simulink model "Roadsense_ScenarioClosedLoopHarness"  (R2025b)
settings: Solver=FixedStepDiscrete  StartTime=0.0  StopTime=25  FixedStep=RsTsBase  RelTol=1e-3
undefined symbols (not defined in the file or in its folder): RsTsBase, RsTsControl, RsTsScenario
settings Model: DataDictionary=Roadsense_Data.sldd  Creator=ragur  LastModifiedBy=ragur

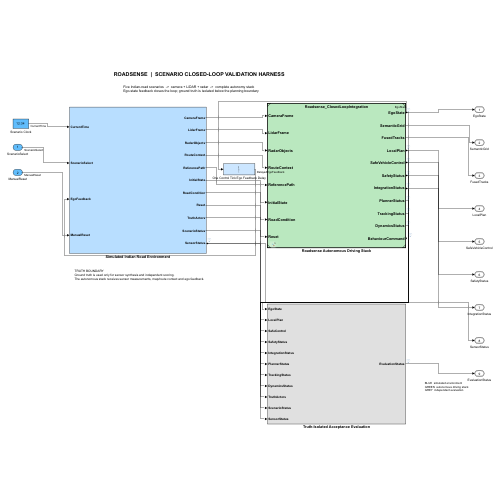
[thumbnail: Simulink's stored preview of the top-level diagram]
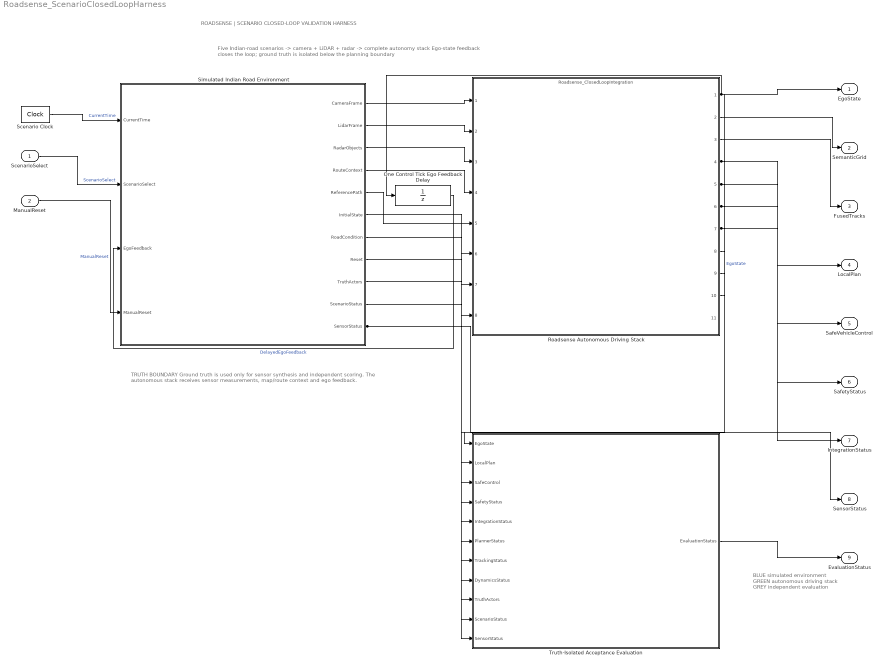
== system Roadsense_ScenarioClosedLoopHarness ==
  note: ROADSENSE | SCENARIO CLOSED-LOOP VALIDATION HARNESS
  note: Five Indian-road scenarios  ->  camera + LiDAR + radar  ->  complete autonomy stack
      | Ego-state feedback closes the loop; ground truth is isolated below the planning boundary
  note: TRUTH BOUNDARY
      | Ground truth is used only for sensor synthesis and independent scoring.
      | The autonomous stack receives sensor measurements, map/route context and ego feedback.
  note: BLUE  simulated environment
      | GREEN  autonomous driving stack
      | GREY  independent evaluation
  ScenarioSelect : Inport  OutDataTypeStr=uint8  SampleTime=RsTsScenario
  ManualReset : Inport  Port=2  OutDataTypeStr=boolean  SampleTime=RsTsControl
  One Control Tick Ego Feedback Delay : UnitDelay  SampleTime=RsTsControl  HasFrameUpgradeWarning=on
  Roadsense Autonomous Driving Stack : ModelReference  ModelNameDialog=Roadsense_ClosedLoopIntegration  SimulationMode=Normal  ModelReferenceVersion=1.1
  Scenario Clock : DigitalClock  SampleTime=RsTsBase
  Simulated Indian Road Environment : Subsystem
  Truth-Isolated Acceptance Evaluation : Subsystem
  EgoState : Outport  OutDataTypeStr=Bus: RsEgoStateBus
  SemanticGrid : Outport  Port=2  OutDataTypeStr=Bus: RsSemanticGridBus
  FusedTracks : Outport  Port=3  OutDataTypeStr=Bus: RsFusedTrackListBus
  LocalPlan : Outport  Port=4  OutDataTypeStr=Bus: RsLocalPlanBus
  SafeVehicleControl : Outport  Port=5  OutDataTypeStr=Bus: RsVehicleControlBus
  SafetyStatus : Outport  Port=6  OutDataTypeStr=Bus: RsSafetyStatusBus
  IntegrationStatus : Outport  Port=7  OutDataTypeStr=Bus: RsIntegrationStatusBus
  SensorStatus : Outport  Port=8  OutDataTypeStr=Bus: RsScenarioSensorStatusBus
  EvaluationStatus : Outport  Port=9  OutDataTypeStr=Bus: RsScenarioEvaluationBus
  wires:
  Scenario Clock/1 -> Simulated Indian Road Environment/1(CurrentTime)  "CurrentTime"
  ScenarioSelect/1 -> Simulated Indian Road Environment/2(ScenarioSelect)  "ScenarioSelect"
  Roadsense Autonomous Driving Stack/1 -> One Control Tick Ego Feedback Delay/1, Truth-Isolated Acceptance Evaluation/1(EgoState), EgoState/1  "EgoState"
  One Control Tick Ego Feedback Delay/1 -> Simulated Indian Road Environment/3(EgoFeedback)  "DelayedEgoFeedback"
  ManualReset/1 -> Simulated Indian Road Environment/4(ManualReset)  "ManualReset"
  Simulated Indian Road Environment/1(CameraFrame) -> Roadsense Autonomous Driving Stack/1
  Simulated Indian Road Environment/2(LidarFrame) -> Roadsense Autonomous Driving Stack/2
  Simulated Indian Road Environment/3(RadarObjects) -> Roadsense Autonomous Driving Stack/3
  Simulated Indian Road Environment/4(RouteContext) -> Roadsense Autonomous Driving Stack/4
  Simulated Indian Road Environment/5(ReferencePath) -> Roadsense Autonomous Driving Stack/5
  Simulated Indian Road Environment/6(InitialState) -> Roadsense Autonomous Driving Stack/6
  Simulated Indian Road Environment/7(RoadCondition) -> Roadsense Autonomous Driving Stack/7
  Simulated Indian Road Environment/8(Reset) -> Roadsense Autonomous Driving Stack/8
  Roadsense Autonomous Driving Stack/4 -> Truth-Isolated Acceptance Evaluation/2(LocalPlan), LocalPlan/1
  Roadsense Autonomous Driving Stack/5 -> Truth-Isolated Acceptance Evaluation/3(SafeControl), SafeVehicleControl/1
  Roadsense Autonomous Driving Stack/6 -> Truth-Isolated Acceptance Evaluation/4(SafetyStatus), SafetyStatus/1
  Roadsense Autonomous Driving Stack/7 -> Truth-Isolated Acceptance Evaluation/5(IntegrationStatus), IntegrationStatus/1
  Roadsense Autonomous Driving Stack/8 -> Truth-Isolated Acceptance Evaluation/6(PlannerStatus)
  Roadsense Autonomous Driving Stack/9 -> Truth-Isolated Acceptance Evaluation/7(TrackingStatus)
  Roadsense Autonomous Driving Stack/10 -> Truth-Isolated Acceptance Evaluation/8(DynamicsStatus)
  Simulated Indian Road Environment/9(TruthActors) -> Truth-Isolated Acceptance Evaluation/9(TruthActors)
  Simulated Indian Road Environment/10(ScenarioStatus) -> Truth-Isolated Acceptance Evaluation/10(ScenarioStatus)
  Simulated Indian Road Environment/11(SensorStatus) -> Truth-Isolated Acceptance Evaluation/11(SensorStatus), SensorStatus/1
  Roadsense Autonomous Driving Stack/2 -> SemanticGrid/1
  Roadsense Autonomous Driving Stack/3 -> FusedTracks/1
  Truth-Isolated Acceptance Evaluation/1(EvaluationStatus) -> EvaluationStatus/1

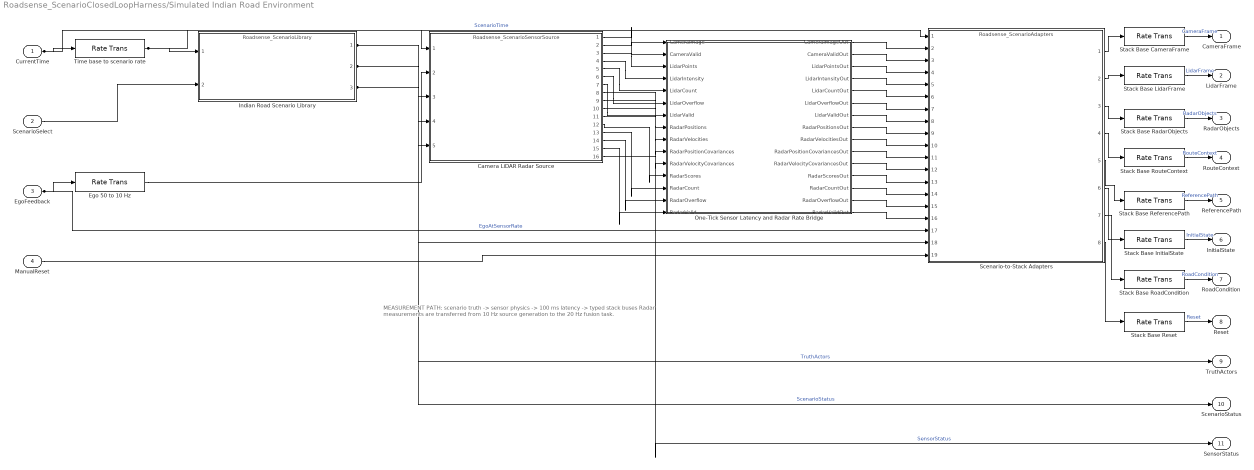
== system Roadsense_ScenarioClosedLoopHarness/Simulated Indian Road Environment ==
  note: MEASUREMENT PATH:  scenario truth -> sensor physics -> 100 ms latency -> typed stack buses
      | Radar measurements are transferred from 10 Hz source generation to the 20 Hz fusion task.
  CurrentTime : Inport  OutDataTypeStr=double  SampleTime=RsTsBase
  ScenarioSelect : Inport  Port=2  OutDataTypeStr=uint8  SampleTime=RsTsScenario
  EgoFeedback : Inport  Port=3  OutDataTypeStr=Bus: RsEgoStateBus  SampleTime=RsTsControl
  ManualReset : Inport  Port=4  OutDataTypeStr=boolean  SampleTime=RsTsControl
  Camera LiDAR Radar Source : ModelReference  ModelNameDialog=Roadsense_ScenarioSensorSource  SimulationMode=Normal  ModelReferenceVersion=1.1
  Ego 50 to 10 Hz : RateTransition  OutPortSampleTime=RsTsScenario
  Indian Road Scenario Library : ModelReference  ModelNameDialog=Roadsense_ScenarioLibrary  SimulationMode=Normal  ModelReferenceVersion=1.1
  One-Tick Sensor Latency and Radar Rate Bridge : Subsystem
  Scenario-to-Stack Adapters : ModelReference  ModelNameDialog=Roadsense_ScenarioAdapters  SimulationMode=Normal  ModelReferenceVersion=1.1
  Stack Base CameraFrame : RateTransition  OutPortSampleTime=RsTsBase
  Stack Base InitialState : RateTransition  OutPortSampleTime=RsTsBase
  Stack Base LidarFrame : RateTransition  OutPortSampleTime=RsTsBase
  Stack Base RadarObjects : RateTransition  OutPortSampleTime=RsTsBase
  Stack Base ReferencePath : RateTransition  OutPortSampleTime=RsTsBase
  Stack Base Reset : RateTransition  OutPortSampleTime=RsTsBase
  Stack Base RoadCondition : RateTransition  OutPortSampleTime=RsTsBase
  Stack Base RouteContext : RateTransition  OutPortSampleTime=RsTsBase
  Time base to scenario rate : RateTransition  OutPortSampleTime=RsTsScenario
  CameraFrame : Outport  OutDataTypeStr=Bus: RsCameraFrameBus
  LidarFrame : Outport  Port=2  OutDataTypeStr=Bus: RsLidarFrameBus
  RadarObjects : Outport  Port=3  OutDataTypeStr=Bus: RsRadarObjectListBus
  RouteContext : Outport  Port=4  OutDataTypeStr=Bus: RsRouteContextBus
  ReferencePath : Outport  Port=5  OutDataTypeStr=Bus: RsReferencePathBus
  InitialState : Outport  Port=6  OutDataTypeStr=Bus: RsEgoStateBus
  RoadCondition : Outport  Port=7  OutDataTypeStr=Bus: RsRoadConditionBus
  Reset : Outport  Port=8  OutDataTypeStr=boolean
  TruthActors : Outport  Port=9  OutDataTypeStr=Bus: RsScenarioActorListBus
  ScenarioStatus : Outport  Port=10  OutDataTypeStr=Bus: RsScenarioStatusBus
  SensorStatus : Outport  Port=11  OutDataTypeStr=Bus: RsScenarioSensorStatusBus
  wires:
  CurrentTime/1 -> Time base to scenario rate/1, Scenario-to-Stack Adapters/1  "ScenarioTime"
  EgoFeedback/1 -> Ego 50 to 10 Hz/1, Scenario-to-Stack Adapters/17  "EgoAtSensorRate"
  Time base to scenario rate/1 -> Indian Road Scenario Library/1, Camera LiDAR Radar Source/1
  ScenarioSelect/1 -> Indian Road Scenario Library/2
  Ego 50 to 10 Hz/1 -> Camera LiDAR Radar Source/2
  Indian Road Scenario Library/2 -> Camera LiDAR Radar Source/3, TruthActors/1  "TruthActors"
  Indian Road Scenario Library/1 -> Camera LiDAR Radar Source/4, Scenario-to-Stack Adapters/18
  Indian Road Scenario Library/3 -> Camera LiDAR Radar Source/5, ScenarioStatus/1  "ScenarioStatus"
  Camera LiDAR Radar Source/1 -> One-Tick Sensor Latency and Radar Rate Bridge/1(CameraImage)
  Camera LiDAR Radar Source/2 -> One-Tick Sensor Latency and Radar Rate Bridge/2(CameraValid)
  Camera LiDAR Radar Source/3 -> One-Tick Sensor Latency and Radar Rate Bridge/3(LidarPoints)
  Camera LiDAR Radar Source/4 -> One-Tick Sensor Latency and Radar Rate Bridge/4(LidarIntensity)
  Camera LiDAR Radar Source/5 -> One-Tick Sensor Latency and Radar Rate Bridge/5(LidarCount)
  Camera LiDAR Radar Source/6 -> One-Tick Sensor Latency and Radar Rate Bridge/6(LidarOverflow)
  Camera LiDAR Radar Source/7 -> One-Tick Sensor Latency and Radar Rate Bridge/7(LidarValid)
  Camera LiDAR Radar Source/8 -> One-Tick Sensor Latency and Radar Rate Bridge/8(RadarPositions)
  Camera LiDAR Radar Source/9 -> One-Tick Sensor Latency and Radar Rate Bridge/9(RadarVelocities)
  Camera LiDAR Radar Source/10 -> One-Tick Sensor Latency and Radar Rate Bridge/10(RadarPositionCovariances)
  Camera LiDAR Radar Source/11 -> One-Tick Sensor Latency and Radar Rate Bridge/11(RadarVelocityCovariances)
  Camera LiDAR Radar Source/12 -> One-Tick Sensor Latency and Radar Rate Bridge/12(RadarScores)
  Camera LiDAR Radar Source/13 -> One-Tick Sensor Latency and Radar Rate Bridge/13(RadarCount)
  Camera LiDAR Radar Source/14 -> One-Tick Sensor Latency and Radar Rate Bridge/14(RadarOverflow)
  Camera LiDAR Radar Source/15 -> One-Tick Sensor Latency and Radar Rate Bridge/15(RadarValid)
  One-Tick Sensor Latency and Radar Rate Bridge/1(CameraImageOut) -> Scenario-to-Stack Adapters/2
  One-Tick Sensor Latency and Radar Rate Bridge/2(CameraValidOut) -> Scenario-to-Stack Adapters/3
  One-Tick Sensor Latency and Radar Rate Bridge/3(LidarPointsOut) -> Scenario-to-Stack Adapters/4
  One-Tick Sensor Latency and Radar Rate Bridge/4(LidarIntensityOut) -> Scenario-to-Stack Adapters/5
  One-Tick Sensor Latency and Radar Rate Bridge/5(LidarCountOut) -> Scenario-to-Stack Adapters/6
  One-Tick Sensor Latency and Radar Rate Bridge/6(LidarOverflowOut) -> Scenario-to-Stack Adapters/7
  One-Tick Sensor Latency and Radar Rate Bridge/7(LidarValidOut) -> Scenario-to-Stack Adapters/8
  One-Tick Sensor Latency and Radar Rate Bridge/8(RadarPositionsOut) -> Scenario-to-Stack Adapters/9
  One-Tick Sensor Latency and Radar Rate Bridge/9(RadarVelocitiesOut) -> Scenario-to-Stack Adapters/10
  One-Tick Sensor Latency and Radar Rate Bridge/10(RadarPositionCovariancesOut) -> Scenario-to-Stack Adapters/11
  One-Tick Sensor Latency and Radar Rate Bridge/11(RadarVelocityCovariancesOut) -> Scenario-to-Stack Adapters/12
  One-Tick Sensor Latency and Radar Rate Bridge/12(RadarScoresOut) -> Scenario-to-Stack Adapters/13
  One-Tick Sensor Latency and Radar Rate Bridge/13(RadarCountOut) -> Scenario-to-Stack Adapters/14
  One-Tick Sensor Latency and Radar Rate Bridge/14(RadarOverflowOut) -> Scenario-to-Stack Adapters/15
  One-Tick Sensor Latency and Radar Rate Bridge/15(RadarValidOut) -> Scenario-to-Stack Adapters/16
  ManualReset/1 -> Scenario-to-Stack Adapters/19
  Scenario-to-Stack Adapters/1 -> Stack Base CameraFrame/1
  Stack Base CameraFrame/1 -> CameraFrame/1  "CameraFrame"
  Scenario-to-Stack Adapters/2 -> Stack Base LidarFrame/1
  Stack Base LidarFrame/1 -> LidarFrame/1  "LidarFrame"
  Scenario-to-Stack Adapters/3 -> Stack Base RadarObjects/1
  Stack Base RadarObjects/1 -> RadarObjects/1  "RadarObjects"
  Scenario-to-Stack Adapters/4 -> Stack Base RouteContext/1
  Stack Base RouteContext/1 -> RouteContext/1  "RouteContext"
  Scenario-to-Stack Adapters/5 -> Stack Base ReferencePath/1
  Stack Base ReferencePath/1 -> ReferencePath/1  "ReferencePath"
  Scenario-to-Stack Adapters/6 -> Stack Base InitialState/1
  Stack Base InitialState/1 -> InitialState/1  "InitialState"
  Scenario-to-Stack Adapters/7 -> Stack Base RoadCondition/1
  Stack Base RoadCondition/1 -> RoadCondition/1  "RoadCondition"
  Scenario-to-Stack Adapters/8 -> Stack Base Reset/1
  Stack Base Reset/1 -> Reset/1  "Reset"
  Camera LiDAR Radar Source/16 -> SensorStatus/1  "SensorStatus"

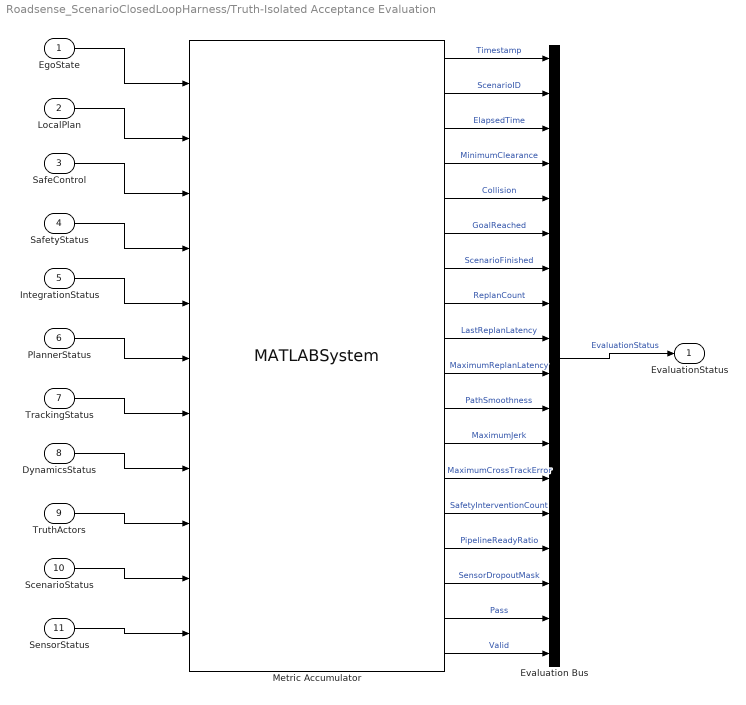
== system Roadsense_ScenarioClosedLoopHarness/Truth-Isolated Acceptance Evaluation ==
  EgoState : Inport  OutDataTypeStr=Bus: RsEgoStateBus
  LocalPlan : Inport  Port=2  OutDataTypeStr=Bus: RsLocalPlanBus
  SafeControl : Inport  Port=3  OutDataTypeStr=Bus: RsVehicleControlBus
  SafetyStatus : Inport  Port=4  OutDataTypeStr=Bus: RsSafetyStatusBus
  IntegrationStatus : Inport  Port=5  OutDataTypeStr=Bus: RsIntegrationStatusBus
  PlannerStatus : Inport  Port=6  OutDataTypeStr=Bus: RsPlannerStatusBus
  TrackingStatus : Inport  Port=7  OutDataTypeStr=Bus: RsTrackingStatusBus
  DynamicsStatus : Inport  Port=8  OutDataTypeStr=Bus: RsVehicleDynamicsStatusBus
  TruthActors : Inport  Port=9  OutDataTypeStr=Bus: RsScenarioActorListBus
  ScenarioStatus : Inport  Port=10  OutDataTypeStr=Bus: RsScenarioStatusBus
  SensorStatus : Inport  Port=11  OutDataTypeStr=Bus: RsScenarioSensorStatusBus
  Evaluation Bus : BusCreator  Inputs=18  OutDataTypeStr=Bus: RsScenarioEvaluationBus
  Metric Accumulator : MATLABSystem  System=RoadsenseScenarioEvaluationSystem  RequiredClearance=RsScenarioMinimumClearance  MaximumAllowedReplanLatency=RsScenarioMaximumReplanLatency  MaximumAllowedPathSmoothness=RsScenarioMaximumPathCurvatureRMS  MaximumAllowedJerk=RsScenarioMaximumJerk  MaximumAllowedCrossTrackError=RsScenarioMaximumCrossTrackError  MinimumReadyRatio=RsScenarioMinimumReadyRatio  SimulateUsing=Interpreted execution
      mask Type: RoadsenseScenarioEvaluationSystem
  EvaluationStatus : Outport  OutDataTypeStr=Bus: RsScenarioEvaluationBus
  wires:
  EgoState/1 -> Metric Accumulator/1
  LocalPlan/1 -> Metric Accumulator/2
  SafeControl/1 -> Metric Accumulator/3
  SafetyStatus/1 -> Metric Accumulator/4
  IntegrationStatus/1 -> Metric Accumulator/5
  PlannerStatus/1 -> Metric Accumulator/6
  TrackingStatus/1 -> Metric Accumulator/7
  DynamicsStatus/1 -> Metric Accumulator/8
  TruthActors/1 -> Metric Accumulator/9
  ScenarioStatus/1 -> Metric Accumulator/10
  SensorStatus/1 -> Metric Accumulator/11
  Metric Accumulator/1 -> Evaluation Bus/1  "Timestamp"
  Metric Accumulator/2 -> Evaluation Bus/2  "ScenarioID"
  Metric Accumulator/3 -> Evaluation Bus/3  "ElapsedTime"
  Metric Accumulator/4 -> Evaluation Bus/4  "MinimumClearance"
  Metric Accumulator/5 -> Evaluation Bus/5  "Collision"
  Metric Accumulator/6 -> Evaluation Bus/6  "GoalReached"
  Metric Accumulator/7 -> Evaluation Bus/7  "ScenarioFinished"
  Metric Accumulator/8 -> Evaluation Bus/8  "ReplanCount"
  Metric Accumulator/9 -> Evaluation Bus/9  "LastReplanLatency"
  Metric Accumulator/10 -> Evaluation Bus/10  "MaximumReplanLatency"
  Metric Accumulator/11 -> Evaluation Bus/11  "PathSmoothness"
  Metric Accumulator/12 -> Evaluation Bus/12  "MaximumJerk"
  Metric Accumulator/13 -> Evaluation Bus/13  "MaximumCrossTrackError"
  Metric Accumulator/14 -> Evaluation Bus/14  "SafetyInterventionCount"
  Metric Accumulator/15 -> Evaluation Bus/15  "PipelineReadyRatio"
  Metric Accumulator/16 -> Evaluation Bus/16  "SensorDropoutMask"
  Metric Accumulator/17 -> Evaluation Bus/17  "Pass"
  Metric Accumulator/18 -> Evaluation Bus/18  "Valid"
  Evaluation Bus/1 -> EvaluationStatus/1  "EvaluationStatus"

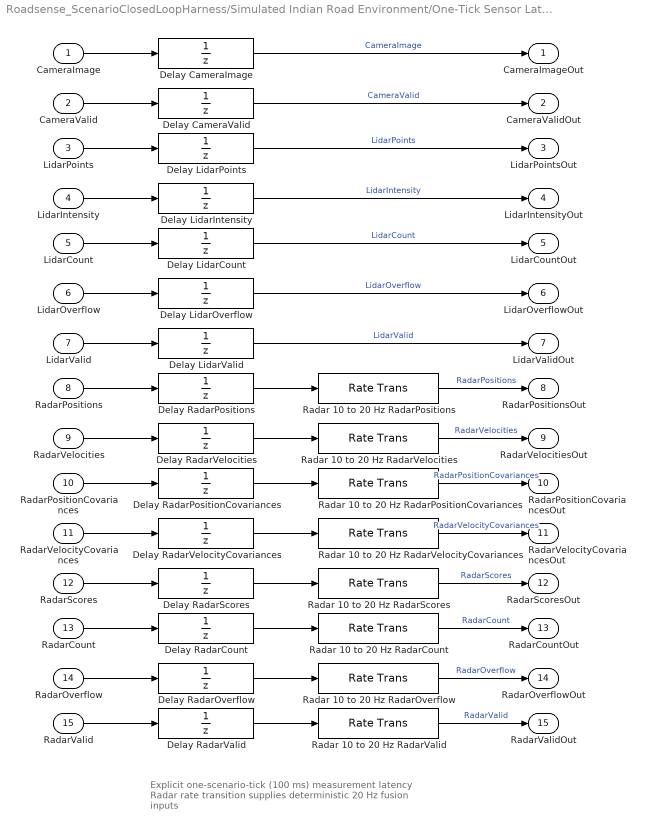
== system Roadsense_ScenarioClosedLoopHarness/Simulated Indian Road Environment/One-Tick Sensor Latency and Radar Rate Bridge ==
  note: Explicit one-scenario-tick (100 ms) measurement latency
      | Radar rate transition supplies deterministic 20 Hz fusion inputs
  CameraImage : Inport  OutDataTypeStr=uint8  PortDimensions=[480 640 3]  SampleTime=RsTsScenario
  CameraValid : Inport  Port=2  OutDataTypeStr=boolean  PortDimensions=1  SampleTime=RsTsScenario
  LidarPoints : Inport  Port=3  OutDataTypeStr=single  PortDimensions=[120000 3]  SampleTime=RsTsScenario
  LidarIntensity : Inport  Port=4  OutDataTypeStr=single  PortDimensions=[120000 1]  SampleTime=RsTsScenario
  LidarCount : Inport  Port=5  OutDataTypeStr=uint32  PortDimensions=1  SampleTime=RsTsScenario
  LidarOverflow : Inport  Port=6  OutDataTypeStr=boolean  PortDimensions=1  SampleTime=RsTsScenario
  LidarValid : Inport  Port=7  OutDataTypeStr=boolean  PortDimensions=1  SampleTime=RsTsScenario
  RadarPositions : Inport  Port=8  OutDataTypeStr=single  PortDimensions=[256 3]  SampleTime=RsTsScenario
  RadarVelocities : Inport  Port=9  OutDataTypeStr=single  PortDimensions=[256 3]  SampleTime=RsTsScenario
  RadarPositionCovariances : Inport  Port=10  OutDataTypeStr=single  PortDimensions=[3 3 256]  SampleTime=RsTsScenario
  RadarVelocityCovariances : Inport  Port=11  OutDataTypeStr=single  PortDimensions=[3 3 256]  SampleTime=RsTsScenario
  RadarScores : Inport  Port=12  OutDataTypeStr=single  PortDimensions=[256 1]  SampleTime=RsTsScenario
  RadarCount : Inport  Port=13  OutDataTypeStr=uint16  PortDimensions=1  SampleTime=RsTsScenario
  RadarOverflow : Inport  Port=14  OutDataTypeStr=boolean  PortDimensions=1  SampleTime=RsTsScenario
  RadarValid : Inport  Port=15  OutDataTypeStr=boolean  PortDimensions=1  SampleTime=RsTsScenario
  Delay CameraImage : UnitDelay  SampleTime=RsTsScenario  HasFrameUpgradeWarning=on
  Delay CameraValid : UnitDelay  SampleTime=RsTsScenario  HasFrameUpgradeWarning=on
  Delay LidarCount : UnitDelay  SampleTime=RsTsScenario  HasFrameUpgradeWarning=on
  Delay LidarIntensity : UnitDelay  SampleTime=RsTsScenario  HasFrameUpgradeWarning=on
  Delay LidarOverflow : UnitDelay  SampleTime=RsTsScenario  HasFrameUpgradeWarning=on
  Delay LidarPoints : UnitDelay  SampleTime=RsTsScenario  HasFrameUpgradeWarning=on
  Delay LidarValid : UnitDelay  SampleTime=RsTsScenario  HasFrameUpgradeWarning=on
  Delay RadarCount : UnitDelay  SampleTime=RsTsScenario  HasFrameUpgradeWarning=on
  Delay RadarOverflow : UnitDelay  SampleTime=RsTsScenario  HasFrameUpgradeWarning=on
  Delay RadarPositionCovariances : UnitDelay  SampleTime=RsTsScenario  HasFrameUpgradeWarning=on
  Delay RadarPositions : UnitDelay  SampleTime=RsTsScenario  HasFrameUpgradeWarning=on
  Delay RadarScores : UnitDelay  SampleTime=RsTsScenario  HasFrameUpgradeWarning=on
  Delay RadarValid : UnitDelay  SampleTime=RsTsScenario  HasFrameUpgradeWarning=on
  Delay RadarVelocities : UnitDelay  SampleTime=RsTsScenario  HasFrameUpgradeWarning=on
  Delay RadarVelocityCovariances : UnitDelay  SampleTime=RsTsScenario  HasFrameUpgradeWarning=on
  Radar 10 to 20 Hz RadarCount : RateTransition  OutPortSampleTime=RsTsFusion
  Radar 10 to 20 Hz RadarOverflow : RateTransition  OutPortSampleTime=RsTsFusion
  Radar 10 to 20 Hz RadarPositionCovariances : RateTransition  OutPortSampleTime=RsTsFusion
  Radar 10 to 20 Hz RadarPositions : RateTransition  OutPortSampleTime=RsTsFusion
  Radar 10 to 20 Hz RadarScores : RateTransition  OutPortSampleTime=RsTsFusion
  Radar 10 to 20 Hz RadarValid : RateTransition  OutPortSampleTime=RsTsFusion
  Radar 10 to 20 Hz RadarVelocities : RateTransition  OutPortSampleTime=RsTsFusion
  Radar 10 to 20 Hz RadarVelocityCovariances : RateTransition  OutPortSampleTime=RsTsFusion
  CameraImageOut : Outport  OutDataTypeStr=uint8  PortDimensions=[480 640 3]
  CameraValidOut : Outport  Port=2  OutDataTypeStr=boolean  PortDimensions=1
  LidarPointsOut : Outport  Port=3  OutDataTypeStr=single  PortDimensions=[120000 3]
  LidarIntensityOut : Outport  Port=4  OutDataTypeStr=single  PortDimensions=[120000 1]
  LidarCountOut : Outport  Port=5  OutDataTypeStr=uint32  PortDimensions=1
  LidarOverflowOut : Outport  Port=6  OutDataTypeStr=boolean  PortDimensions=1
  LidarValidOut : Outport  Port=7  OutDataTypeStr=boolean  PortDimensions=1
  RadarPositionsOut : Outport  Port=8  OutDataTypeStr=single  PortDimensions=[256 3]
  RadarVelocitiesOut : Outport  Port=9  OutDataTypeStr=single  PortDimensions=[256 3]
  RadarPositionCovariancesOut : Outport  Port=10  OutDataTypeStr=single  PortDimensions=[3 3 256]
  RadarVelocityCovariancesOut : Outport  Port=11  OutDataTypeStr=single  PortDimensions=[3 3 256]
  RadarScoresOut : Outport  Port=12  OutDataTypeStr=single  PortDimensions=[256 1]
  RadarCountOut : Outport  Port=13  OutDataTypeStr=uint16  PortDimensions=1
  RadarOverflowOut : Outport  Port=14  OutDataTypeStr=boolean  PortDimensions=1
  RadarValidOut : Outport  Port=15  OutDataTypeStr=boolean  PortDimensions=1
  wires:
  CameraImage/1 -> Delay CameraImage/1
  Delay CameraImage/1 -> CameraImageOut/1  "CameraImage"
  CameraValid/1 -> Delay CameraValid/1
  Delay CameraValid/1 -> CameraValidOut/1  "CameraValid"
  LidarPoints/1 -> Delay LidarPoints/1
  Delay LidarPoints/1 -> LidarPointsOut/1  "LidarPoints"
  LidarIntensity/1 -> Delay LidarIntensity/1
  Delay LidarIntensity/1 -> LidarIntensityOut/1  "LidarIntensity"
  LidarCount/1 -> Delay LidarCount/1
  Delay LidarCount/1 -> LidarCountOut/1  "LidarCount"
  LidarOverflow/1 -> Delay LidarOverflow/1
  Delay LidarOverflow/1 -> LidarOverflowOut/1  "LidarOverflow"
  LidarValid/1 -> Delay LidarValid/1
  Delay LidarValid/1 -> LidarValidOut/1  "LidarValid"
  RadarPositions/1 -> Delay RadarPositions/1
  Delay RadarPositions/1 -> Radar 10 to 20 Hz RadarPositions/1
  Radar 10 to 20 Hz RadarPositions/1 -> RadarPositionsOut/1  "RadarPositions"
  RadarVelocities/1 -> Delay RadarVelocities/1
  Delay RadarVelocities/1 -> Radar 10 to 20 Hz RadarVelocities/1
  Radar 10 to 20 Hz RadarVelocities/1 -> RadarVelocitiesOut/1  "RadarVelocities"
  RadarPositionCovariances/1 -> Delay RadarPositionCovariances/1
  Delay RadarPositionCovariances/1 -> Radar 10 to 20 Hz RadarPositionCovariances/1
  Radar 10 to 20 Hz RadarPositionCovariances/1 -> RadarPositionCovariancesOut/1  "RadarPositionCovariances"
  RadarVelocityCovariances/1 -> Delay RadarVelocityCovariances/1
  Delay RadarVelocityCovariances/1 -> Radar 10 to 20 Hz RadarVelocityCovariances/1
  Radar 10 to 20 Hz RadarVelocityCovariances/1 -> RadarVelocityCovariancesOut/1  "RadarVelocityCovariances"
  RadarScores/1 -> Delay RadarScores/1
  Delay RadarScores/1 -> Radar 10 to 20 Hz RadarScores/1
  Radar 10 to 20 Hz RadarScores/1 -> RadarScoresOut/1  "RadarScores"
  RadarCount/1 -> Delay RadarCount/1
  Delay RadarCount/1 -> Radar 10 to 20 Hz RadarCount/1
  Radar 10 to 20 Hz RadarCount/1 -> RadarCountOut/1  "RadarCount"
  RadarOverflow/1 -> Delay RadarOverflow/1
  Delay RadarOverflow/1 -> Radar 10 to 20 Hz RadarOverflow/1
  Radar 10 to 20 Hz RadarOverflow/1 -> RadarOverflowOut/1  "RadarOverflow"
  RadarValid/1 -> Delay RadarValid/1
  Delay RadarValid/1 -> Radar 10 to 20 Hz RadarValid/1
  Radar 10 to 20 Hz RadarValid/1 -> RadarValidOut/1  "RadarValid"
